simulink model "saturation_and_dynamic_saturation"  (R2021a)
settings: Solver=VariableStepAuto  StartTime=0.0  StopTime=10.0  RelTol=1e-3
libraries: simulink x1
settings Model: Creator=DELL  LastModifiedBy=DELL

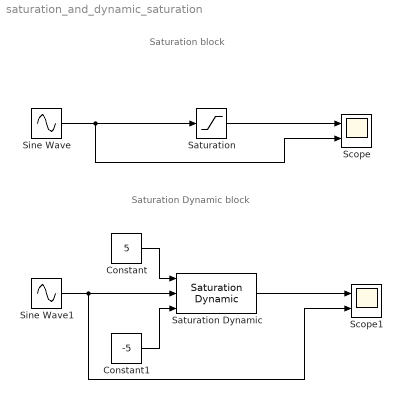
== system saturation_and_dynamic_saturation ==
  note: Saturation block
  note: Saturation Dynamic block
  Constant : Constant  Value=5
  Constant1 : Constant  Value=-5
  Saturation : Saturate  UpperLimit=5  LowerLimit=-5
  Saturation Dynamic : simulink/Discontinuities/Saturation Dynamic  OutMin=[]  OutMax=[]  OutDataTypeStr=Inherit: Same as second input  OutDataType=fixdt(1, 16)  OutScaling=2^-10  DoSatur=off
  Scope : Scope  NumInputPorts=2
  Scope1 : Scope  NumInputPorts=2
  Sine Wave : Sin  Amplitude=10  SampleTime=0
  Sine Wave1 : Sin  Amplitude=10  SampleTime=0
  wires:
  Sine Wave/1 -> Scope/2, Saturation/1
  Saturation/1 -> Scope/1
  Sine Wave1/1 -> Scope1/2, Saturation Dynamic/2
  Constant/1 -> Saturation Dynamic/1
  Constant1/1 -> Saturation Dynamic/3
  Saturation Dynamic/1 -> Scope1/1
